simulink subsystem "tiltAngleKalman"  (R2024a)
settings: Solver=VariableStepAuto  StartTime=0.0  StopTime=10.0  RelTol=1e-3
undefined symbols (not defined in the file or in its folder): angleEstRate, Q_ang_kf, R_ang_kf
settings Model: Creator=Peter  LastModifiedBy=Peter

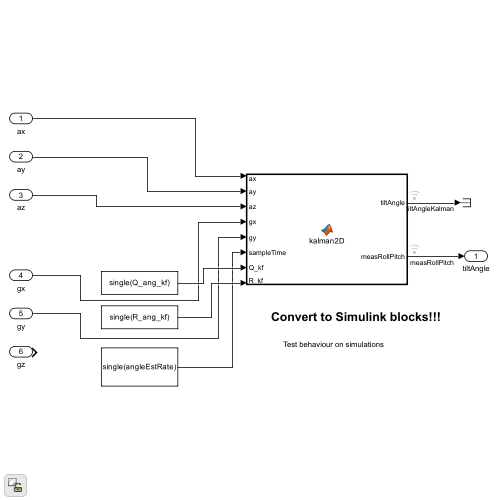
[thumbnail: Simulink's stored preview of the top-level diagram]
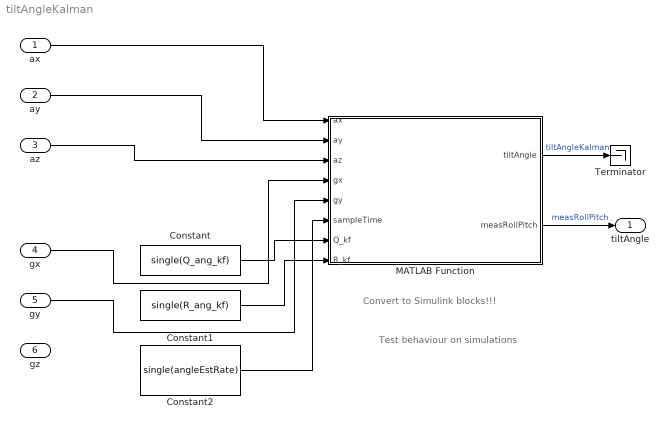
== system tiltAngleKalman ==
  note: Test behaviour on simulations
  note: Convert to Simulink blocks!!!
  ax : Inport
  ay : Inport  Port=2
  az : Inport  Port=3
  gx : Inport  Port=4
  gy : Inport  Port=5
  gz : Inport  Port=6
  Constant : Constant  Value=single(Q_ang_kf)  OutDataTypeStr=single
  Constant1 : Constant  Value=single(R_ang_kf)  OutDataTypeStr=single
  Constant2 : Constant  Value=single(angleEstRate)  OutDataTypeStr=single
  MATLAB Function : MATLAB Function  TreatAsAtomicUnit=on
  Terminator : Terminator
  tiltAngle : Outport
  wires:
  ax/1 -> MATLAB Function/1(ax)
  ay/1 -> MATLAB Function/2(ay)
  az/1 -> MATLAB Function/3(az)
  gx/1 -> MATLAB Function/4(gx)
  gy/1 -> MATLAB Function/5(gy)
  MATLAB Function/1(tiltAngle) -> Terminator/1  "tiltAngleKalman"
  Constant2/1 -> MATLAB Function/6(sampleTime)
  Constant/1 -> MATLAB Function/7(Q_kf)
  Constant1/1 -> MATLAB Function/8(R_kf)
  MATLAB Function/2(measRollPitch) -> tiltAngle/1  "measRollPitch"

== matlab function tiltAngleKalman/MATLAB Function ==
  data: ax input single; tiltAngle output single; ay input single; az input single; gx input single; gy input single; sampleTime input single; Q_kf input single; R_kf input single; measRollPitch output single
function [tiltAngle,measRollPitch] = kalman2D(ax, ay, az, gx, gy,sampleTime,Q_kf,R_kf)
%#codegen

persistent x P instance

dt = single(sampleTime); % Sample time
deg2rad = single(pi / 180);

% Initialize persistent state vector and covariance matrix
if isempty(instance)
    % State: [theta_x; theta_y; omega_x; omega_y]
    x = single(zeros(4, 1));
    P = single(eye(4) * 0.1);
    instance = true;
end

% System dynamics matrix
A = single([1 0 dt 0;
             0 1 0 dt;
             0 0 1  0;
             0 0 0  1]);

% Process noise covariance (tune as needed)
Q = single(Q_kf);

% Measurement matrix: we only measure [theta_x, theta_y]
H = single([1 0 0 0;
            0 1 0 0]);

% Measurement noise covariance
R = single(R_kf);

% ====== PREDICT STEP ======

% Inject new gyro measurements into angular rate state (rad/s)!!!!!!!!!!!!
x(3) = gy * deg2rad;
x(4) = gx * deg2rad;

% Can be:
   % B = single([0 0;
   %              0 0;
   %              1 0;
   %              0 1]);
   % 
   %  % ===== PREDICT STEP =====
   %  % Gyro control input (rad/s)
   %  u = [gx; gy] * deg2rad;
   % 
   %  % Predict next state
   %  x = A * x + B * u;

% Predict state and covariance
x = A * x;
P = A * P * A' + Q;

% ====== MEASUREMENT FROM ACCELEROMETER ======

% Estimate roll and pitch from accelerometer
roll_meas  = atan2(ax,az);
% pitch_meas = atan(-ax / sqrt(ay^2 + az^2));
pitch_meas = atan2(ay,az);
z = [roll_meas; pitch_meas];

measRollPitch = z;


% ====== UPDATE STEP ======
K = P * H' / (H * P * H' + R);
x = x + K * (z - H * x);
P = (eye(4) - K * H) * P;

% Output estimated [roll; pitch]
tiltAngle = x(1:2);
end
